simulink model "Part1_2"  (R2017a)
settings: Solver=VariableStepAuto  StartTime=0.0  StopTime=10.0  RelTol=1e-3
libraries: commchan3 x1, commrandsrc3 x1, commsink2 x1, dspsigops x1
settings Model: Creator=mhuynh7  LastModifiedBy=mhuynh7

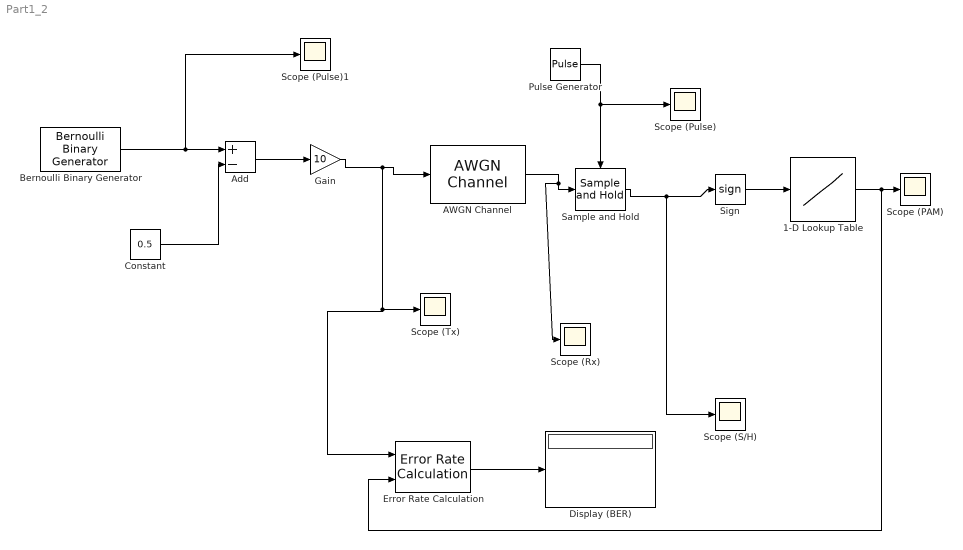
== system Part1_2 ==
  1-D Lookup Table : Lookup_n-D  NumberOfTableDimensions=1  BreakpointsForDimension1=[-1,0,1]  Table=[-5,-5,5]  InternalRulePriority=Speed  RndMeth=Simplest  InputSameDT=on
  AWGN Channel : commchan3/AWGN Channel  InputProcessing=Columns as channels (frame based)  seed=randseed  noiseMode="Signal to noise ratio  (Eb/No)"  EbNodB=10  EsNodB=10  SNRdB=10  bitsPerSym=1  Ps=25  Tsym=0.001  variance=1
  Add : Sum  Inputs=+-
  Bernoulli Binary Generator : commrandsrc3/Bernoulli Binary Generator  ProbabilityOfZero=0.5  SeedSource=Auto  Seed=0  SampleTime=0.001  SamplesPerFrame=1  OutputDataType=double  SimulateUsing=Interpreted execution
  Constant : Constant  Value=0.5
  Display (BER) : Display
  Error Rate Calculation : commsink2/Error Rate Calculation  N=1  st_delay=0  cp_mode=Entire frame  subframe=[]  PMode=Port  WsName=ErrorVec  RsMode2=off  stop=off  numErr=100  maxBits=1e6
  Gain : Gain  Gain=10
  Pulse Generator : DiscretePulseGenerator  PhaseDelay=1  SampleTime=0.5e-3
  Sample and Hold : dspsigops/Sample and Hold  trig=Rising edge  initCond=0  latchinput=off
  Scope (PAM) : Scope
  Scope (Pulse) : Scope
  Scope (Pulse)1 : Scope
  Scope (Rx) : Scope
  Scope (S/H) : Scope
  Scope (Tx) : Scope
  Sign : Signum
  wires:
  Constant/1 -> Add/2
  Bernoulli Binary Generator/1 -> Scope (Pulse)1/1, Add/1
  Add/1 -> Gain/1
  Gain/1 -> Error Rate Calculation/1, Scope (Tx)/1, AWGN Channel/1
  AWGN Channel/1 -> Scope (Rx)/1, Sample and Hold/1
  Sample and Hold/1 -> Scope (S/H)/1, Sign/1
  Sign/1 -> 1-D Lookup Table/1
  1-D Lookup Table/1 -> Error Rate Calculation/2, Scope (PAM)/1
  Pulse Generator/1 -> Scope (Pulse)/1, Sample and Hold/Trigger
  Error Rate Calculation/1 -> Display (BER)/1
